simulink model "W01_openloop"  (R2024b)
settings: Solver=ode4  StartTime=0  StopTime=T_final  FixedStep=h  RelTol=1e-3
StopFcn:
  | W01_plot;
values from neighbouring files (symbols this model uses):
  animate = 1    [W01_0_setup.m]    (also in W01_setup.m)
  beta_c = 0    [W01_0_setup.m]    (also in W01_setup.m)
  dn = 3.5    [W01_0_setup.m]    (also in W01_F_button_check.m = str2double(get_param([m '/Drive command/dn'], 'Value')); W01_setup.m)
  h = 0.02    [W01_0_setup.m]    (also in W01_1_build_openloop.m = Simulink.Annotation([m '/note']); W01_E_build_current.m = Simulink.Annotation([sub '/note']); W01_F_build_interactive.m = Simulink.Annotation([m '/note']); W01_G_build_rc.m = Simulink.Annotation([m '/note']))
  mp = 25    [W01_0_setup.m]    (also in W01_setup.m)
  n0 = 60    [W01_0_setup.m]    (also in W01_F_button_check.m = str2double(get_param([m '/Drive command/n0'], 'Value')); W01_setup.m)
  rp = [0.05 0 -0.35]'    [W01_0_setup.m]    (also in W01_setup.m)
  t_phase = [30 60 90 120]    [W01_0_setup.m]    (also in W01_setup.m)
  V_c = 0    [W01_0_setup.m]    (also in W01_setup.m)
  x0 = zeros(12,1)    [W01_0_setup.m]    (also in W01_E_current_run.m = L0(1) + 16; W01_setup.m)
settings Model: Creator=admin  LastModifiedBy=wkyou
settings DataIOCC: ReturnWorkspaceOutputs=off

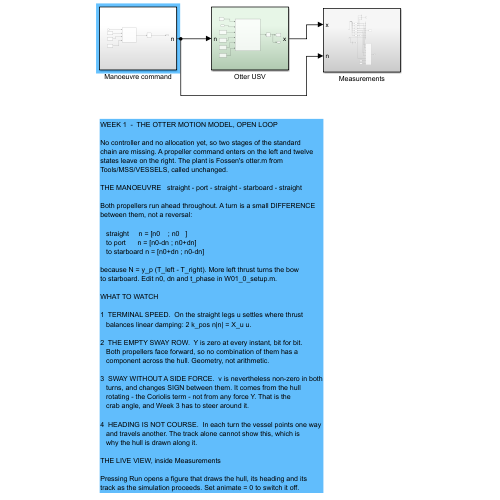
[thumbnail: Simulink's stored preview of the top-level diagram]
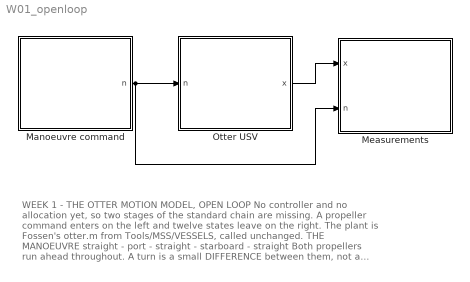
== system W01_openloop ==
  note: WEEK 1  -  THE OTTER MOTION MODEL, OPEN LOOP
      |
      | No controller and no allocation yet, so two stages of the standard
      | chain are missing. A propeller command enters on the left and twelve
      | states leave on the right. The plant is Fossen's otter.m from
      | Tools/MSS/VESSELS, called unchanged.
      |
      | THE MANOEUVRE   straight - port - straight - starboard - straight
      |
      | Both propellers run ahead throughout. A turn is a small DIFFERENCE
      | between them, not a reversal:
      |
      |    straight     n = [n0    ; n0   ]
      |    to port      n = [n0-dn ; n0+dn]
      |    to starboard n = [n0+dn ; n0-dn]
      |
      | because N = y_p (T_left - T_right). More left thrust turns the bow
      | to starboard. Edit n0, dn and t_phase in W01_0_setup.m.
      |
      | WHAT TO WATCH
      |
      | 1  TERMINAL SPEED.  On the straight legs u settles where thrust
      |    balances linear damping: 2 k_pos n|n| = X_u u.
      |
      | 2  THE EMPTY SWAY ROW.  Y is zero at every instant, bit for bit.
      |    Both propellers face forward, so no combination of them has a
      |    component across the hull. Geometry, not arithmetic.
      |
      | 3  SWAY WITHOUT A SIDE FORCE.  v is nevertheless non-zero in both
      |    turns, and changes SIGN between them. It comes from the hull
      |    rotating - the Coriolis term - not from any force Y. That is the
      |    crab angle, and Week 3 has to steer around it.
      |
      | 4  HEADING IS NOT COURSE.  In each turn the vessel points one way
      |    and travels another. The track alone cannot show this, which is
      |    why the hull is drawn along it.
      |
      | THE LIVE VIEW, inside Measurements
      |
      | Pressing Run opens a figure that draws the hull, its heading and its
      | track as the simulation proceeds. Set animate = 0 to switch it off.
  Manoeuvre command : Subsystem
  Measurements : Subsystem
  Otter USV : Subsystem
  wires:
  Manoeuvre command/1(n) -> Otter USV/1(n), Measurements/2(n)
  Otter USV/1(x) -> Measurements/1(x)

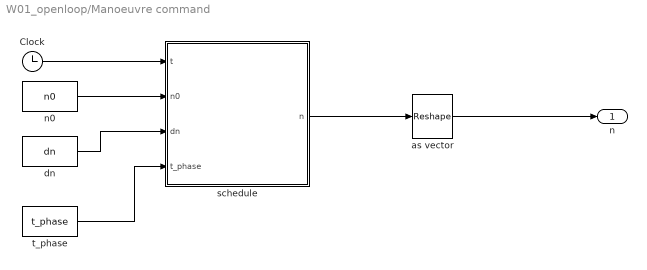
== system W01_openloop/Manoeuvre command ==
  Clock : Clock
  as vector : Reshape
  dn : Constant  Value=dn
  n0 : Constant  Value=n0
  schedule : MATLAB Function  TreatAsAtomicUnit=on
  t_phase : Constant  Value=t_phase
  n : Outport
  wires:
  Clock/1 -> schedule/1(t)
  n0/1 -> schedule/2(n0)
  dn/1 -> schedule/3(dn)
  t_phase/1 -> schedule/4(t_phase)
  schedule/1(n) -> as vector/1
  as vector/1 -> n/1

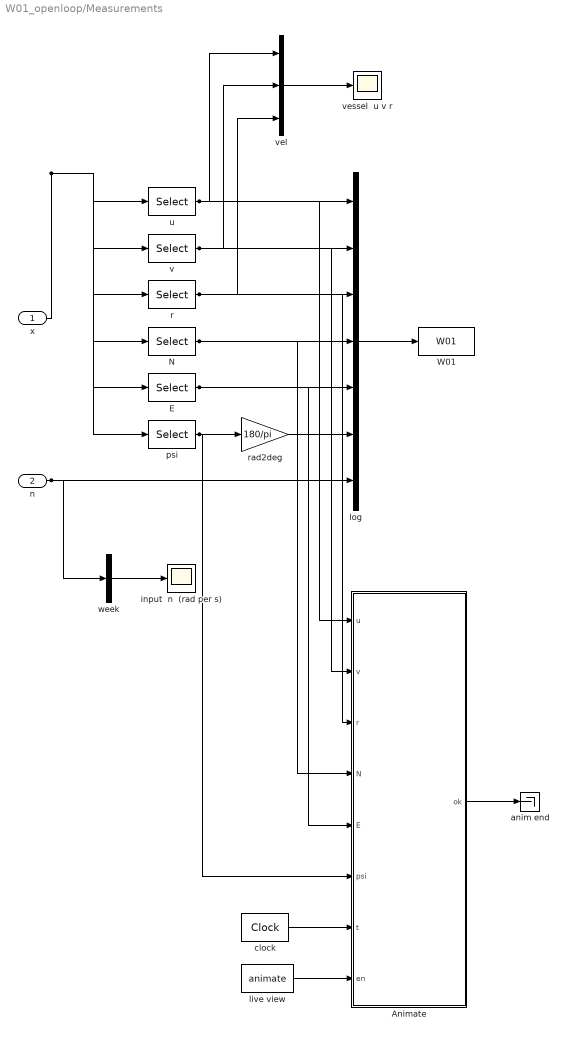
== system W01_openloop/Measurements ==
  x : Inport
  n : Inport  Port=2
  Animate : MATLAB Function  TreatAsAtomicUnit=on
  E : Selector  InputPortWidth=12  IndexOptions=Index vector (dialog)  Indices=8  OutputSizes=1
  N : Selector  InputPortWidth=12  IndexOptions=Index vector (dialog)  Indices=7  OutputSizes=1
  W01 : ToWorkspace  VariableName=W01  SaveFormat=Structure With Time  SampleTime=-1
  anim end : Terminator
  clock : DigitalClock  SampleTime=h
  input  n  (rad per s) : Scope
  live view : Constant  Value=animate
  log : Mux  Inputs=7
  psi : Selector  InputPortWidth=12  IndexOptions=Index vector (dialog)  Indices=12  OutputSizes=1
  r : Selector  InputPortWidth=12  IndexOptions=Index vector (dialog)  Indices=6  OutputSizes=1
  rad2deg : Gain  Gain=180/pi
  u : Selector  InputPortWidth=12  IndexOptions=Index vector (dialog)  Indices=1  OutputSizes=1
  v : Selector  InputPortWidth=12  IndexOptions=Index vector (dialog)  Indices=2  OutputSizes=1
  vel : Mux  Inputs=3
  vessel  u v r : Scope
  week : Mux  Inputs=1
  wires:
  x/1 -> u/1, v/1, r/1, N/1, E/1, psi/1
  log/1 -> W01/1
  psi/1 -> rad2deg/1, Animate/6(psi)
  u/1 -> log/1, vel/1, Animate/1(u)
  v/1 -> log/2, vel/2, Animate/2(v)
  r/1 -> log/3, vel/3, Animate/3(r)
  N/1 -> log/4, Animate/4(N)
  E/1 -> log/5, Animate/5(E)
  rad2deg/1 -> log/6
  n/1 -> log/7, week/1
  vel/1 -> vessel  u v r/1
  week/1 -> input  n  (rad per s)/1
  clock/1 -> Animate/7(t)
  live view/1 -> Animate/8(en)
  Animate/1(ok) -> anim end/1

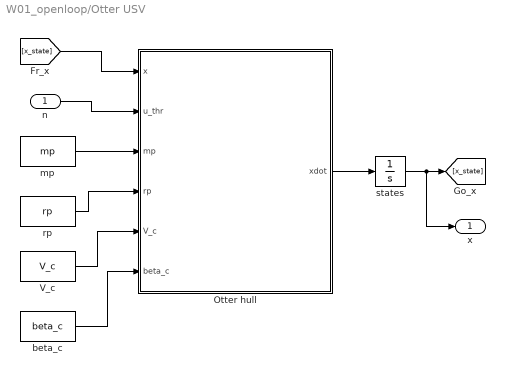
== system W01_openloop/Otter USV ==
  n : Inport
  Otter hull : MATLAB Function  TreatAsAtomicUnit=on
  V_c : Constant  Value=V_c
  beta_c : Constant  Value=beta_c
  mp : Constant  Value=mp
  rp : Constant  Value=rp
  states : Integrator  InitialCondition=x0
  x : Outport
  wires:
  states/1 -> [x_state], x/1
  [x_state] -> Otter hull/1(x)
  beta_c/1 -> Otter hull/6(beta_c)
  V_c/1 -> Otter hull/5(V_c)
  rp/1 -> Otter hull/4(rp)
  mp/1 -> Otter hull/3(mp)
  n/1 -> Otter hull/2(u_thr)
  Otter hull/1(xdot) -> states/1

== matlab function W01_openloop/Otter USV/Otter hull ==
  data: x input; xdot output double size=[12 1]; u_thr input; mp input; rp input; V_c input; beta_c input
function xdot = otter_hull(x, u_thr, mp, rp, V_c, beta_c)
% Fossen's otter.m, called unchanged from Tools/MSS/VESSELS.
%
%   x       12 states, fed back from the integrator
%   u_thr   propeller shaft speeds [rad/s]
%
% otter.m is not written for code generation, so the call is extrinsic and
% xdot has to be pre-sized for Simulink to know the output width.
coder.extrinsic('otter');

xdot = zeros(12,1);
xdot = otter(x, u_thr, mp, rp, V_c, beta_c);
end

== matlab function W01_openloop/Manoeuvre command/schedule ==
  data: t input; n output double size=[2 1]; n0 input; dn input; t_phase input
function n = schedule(t, n0, dn, t_phase)
%#codegen
%SCHEDULE  Propeller command as a function of time.
%
%    straight -> port -> straight -> starboard -> straight
%
%  Both propellers stay ahead the whole time - nothing is ever reversed.
%  A turn is a small DIFFERENCE between the two shaft speeds, because the
%  yaw moment is N = y_p (T_left - T_right). More thrust on the left turns
%  the bow to starboard, so a PORT turn slows the LEFT propeller.
%
%  dn = 0 gives a constant command, which is what the terminal-speed sweep
%  in section C uses.

nL = n0;  nR = n0;
if t >= t_phase(1) && t < t_phase(2)
    nL = n0 + dn;   nR = n0 - dn;      % port      (bow swings to -psi)
elseif t >= t_phase(3) && t < t_phase(4)
    nL = n0 - dn;   nR = n0 + dn;      % starboard (bow swings to +psi)
end
n = [nL; nR];

== matlab function W01_openloop/Measurements/Animate ==
  data: u input; ok output; v input; r input; N input; E input; psi input; t input; en input
function ok = Animate(u, v, r, N, E, psi, t, en)
%#codegen
% Live view of the vessel while the model runs.
%
% A MATLAB Function block cannot plot, so the drawing function is declared
% extrinsic: Simulink calls plain MATLAB rather than generating code for it.
% Set animate = 0 in the setup script to switch the live view off.
%
% psi arrives in RADIANS and r in rad/s - the units otter.m works in. The
% wrapper converts them for display, in one place, so no two figures in the
% course can disagree about what a degree is.
coder.extrinsic('W01_animate');
ok = 1;
if en > 0.5
    W01_animate(u, v, r, N, E, psi, t);
end
end
